simulink model "test_s_function"  (R2024a)
settings: Solver=ode4  StartTime=0.0  StopTime=Inf  FixedStep=1e-3  RelTol=1e-3
settings Model: Creator=sdcnlab  LastModifiedBy=sdcnlab
settings RTWCC: CustomSource=/home/sdcnlab/Desktop/s-function/src/s_function.cpp /home/sdcnlab/Desktop/s-function/src/optical_flow_velocity.cpp  CustomLibrary=/usr/local/lib/libopencv_calib3d.so;/usr/local/lib/libopencv_core.so;/usr/local/lib/libopencv_dnn.so;/usr/local/lib/libopencv_features2d.so;/usr/local/lib/libopencv_flann.so;/usr/local/lib/libopencv_gapi.so;/usr/local/lib/libopencv_highgui.so;/usr/local/lib/libopencv_imgcodecs.so;/usr/local/lib/libopencv_imgproc.so;/usr/local/lib/libopencv_ml.so;/usr/local/lib/libopencv_objdetect.so;/usr/local/lib/libopencv_photo.so;/usr/local/lib/libopencv_stitching.so;/usr/local/lib/libopencv_video.so;/usr/local/lib/libopencv_videoio.so
settings RTWCC: CustomInclude=|
  | /home/sdcnlab/Desktop/s-function/include;/usr/local/include/opencv4
  | /usr/local/lib

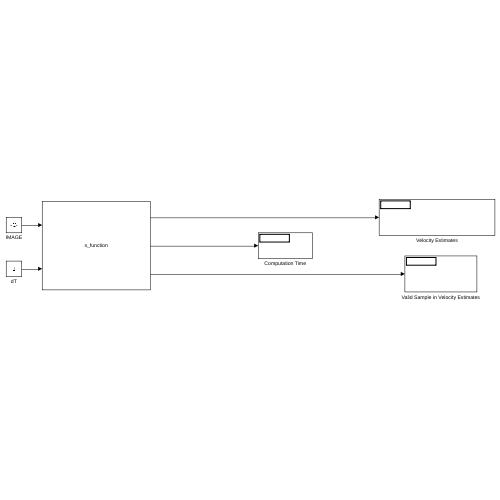
[thumbnail: Simulink's stored preview of the top-level diagram]
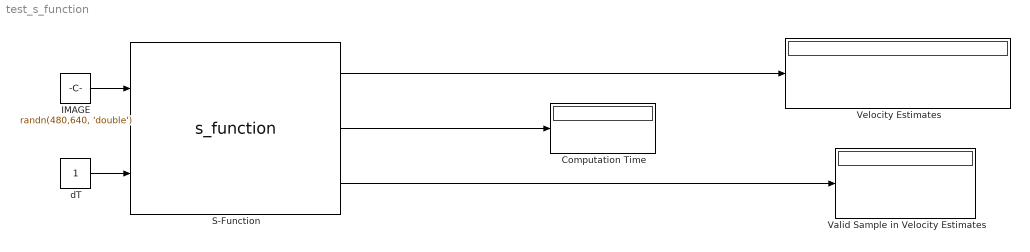
== system test_s_function ==
  Computation Time : Display
  IMAGE : Constant  Value=randn(480,640, 'double')
  S-Function : S-Function  FunctionName=s_function  Parameters=2e-3,1280,1280,1,480,640  SFunctionDeploymentMode=off  EnableBusSupport=off
  Valid Sample in Velocity Estimates : Display
  Velocity Estimates : Display
  dT : Constant
  wires:
  dT/1 -> S-Function/2
  IMAGE/1 -> S-Function/1
  S-Function/1 -> Velocity Estimates/1
  S-Function/3 -> Valid Sample in Velocity Estimates/1
  S-Function/2 -> Computation Time/1
